simulink model "SIMULINK_LQR"  (R2020a)
settings: Solver=VariableStepAuto  StartTime=0.0  StopTime=40  FixedStep=0.1  RelTol=1e-3
settings Model: Creator=CepaTech  LastModifiedBy=CepaTech

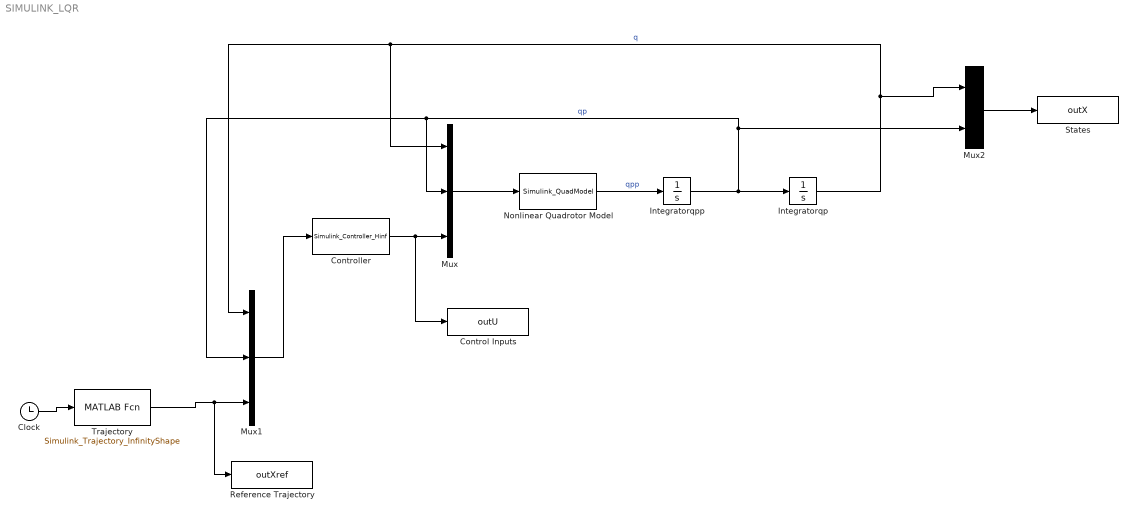
== system SIMULINK_LQR ==
  Clock : Clock
  Control Inputs : ToWorkspace  VariableName=outU  SampleTime=-1
  Controller : MATLABFcn  MATLABFcn=Simulink_Controller_Hinf
  Integratorqp : Integrator  InitialCondition=[8;0;0;0;0;0]
  Integratorqpp : Integrator  InitialCondition=[0;0;0;0;0;0]
  Mux : Mux  Inputs=3
  Mux1 : Mux  Inputs=3
  Mux2 : Mux  Inputs=2
  Nonlinear Quadrotor Model : MATLABFcn  MATLABFcn=Simulink_QuadModel
  Reference Trajectory : ToWorkspace  VariableName=outXref  SampleTime=-1
  States : ToWorkspace  VariableName=outX  SampleTime=-1
  Trajectory : MATLABFcn  MATLABFcn=Simulink_Trajectory_InfinityShape
  wires:
  Mux/1 -> Nonlinear Quadrotor Model/1
  Nonlinear Quadrotor Model/1 -> Integratorqpp/1  "qpp"
  Integratorqpp/1 -> Mux2/2, Mux1/2, Mux/2, Integratorqp/1  "qp"
  Integratorqp/1 -> Mux2/1, Mux1/1, Mux/1  "q"
  Mux1/1 -> Controller/1
  Trajectory/1 -> Reference Trajectory/1, Mux1/3
  Clock/1 -> Trajectory/1
  Controller/1 -> Control Inputs/1, Mux/3
  Mux2/1 -> States/1
